simulink model "robot_ctc"  (R2019b)
settings: Solver=FixedStepAuto  StartTime=0.0  StopTime=20  FixedStep=0.001  RelTol=1e-3
InitFcn:
  | l1 = 0.26;
  | l2 = 0.26;
  | lc1 = 0.0983;
  | lc2 = 0.0229;
  | m1 = 6.5225;
  | m2 = 2.0458;
  | I1 = 0.1213;
  | I2 = 0.0116;
  | g = 9.81;
  | 
  | q0 = [pi/2, pi/6];
  | dq0 = [0, 0];
  | 
  | Kv = [10, 0; 0, 10];
  | Kp = [10, 0; 0, 10];
settings Model: Creator=jgakl

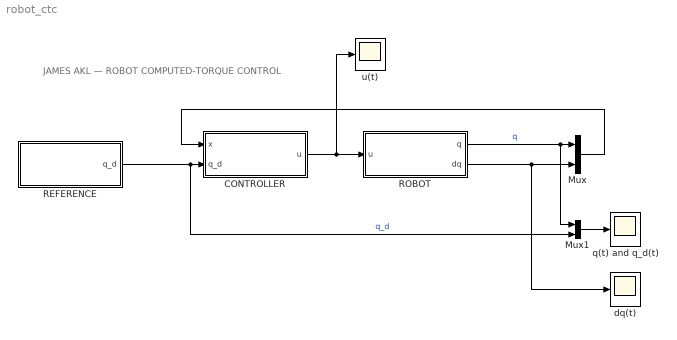
== system robot_ctc ==
  note: JAMES AKL — ROBOT COMPUTED-TORQUE CONTROL
  CONTROLLER : Subsystem
  Mux : Mux  Inputs=2
  Mux1 : Mux  Inputs=2
  REFERENCE : Subsystem
  ROBOT : Subsystem
  dq(t) : Scope
  q(t) and q_d(t) : Scope
  u(t) : Scope
  wires:
  CONTROLLER/1(u) -> u(t)/1, ROBOT/1(u)
  ROBOT/1(q) -> Mux1/1, Mux/1  "q"
  ROBOT/2(dq) -> dq(t)/1, Mux/2
  Mux/1 -> CONTROLLER/1(x)
  REFERENCE/1(q_d) -> CONTROLLER/2(q_d), Mux1/2  "q_d"
  Mux1/1 -> q(t) and q_d(t)/1

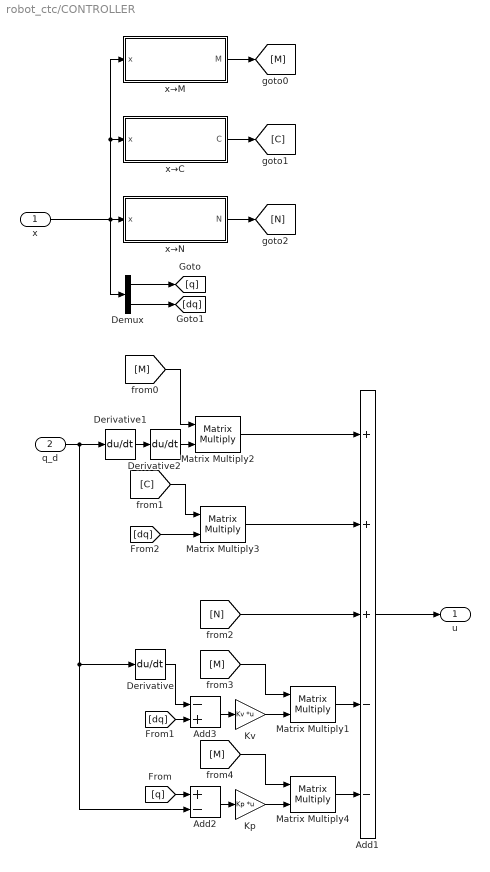
== system robot_ctc/CONTROLLER ==
  x : Inport
  q_d : Inport  Port=2
  Add1 : Sum  Inputs=+++--
  Add2 : Sum  Inputs=+-
  Add3 : Sum  Inputs=-+
  Demux : Demux  Outputs=2
  Derivative : Derivative
  Derivative1 : Derivative
  Derivative2 : Derivative
  Kp : Gain  Gain=Kp  Multiplication=Matrix(K*u) (u vector)
  Kv : Gain  Gain=Kv  Multiplication=Matrix(K*u) (u vector)
  Matrix Multiply{1..4} (4 alike) : Product  Multiplication=Matrix(*)
  x→C : Subsystem
  x→M : Subsystem
  x→N : Subsystem
  u : Outport
  wires:
  x→N/1(N) -> [N]
  x→C/1(C) -> [C]
  x/1 -> x→M/1(x), x→C/1(x), x→N/1(x), Demux/1
  x→M/1(M) -> [M]
  q_d/1 -> Derivative1/1, Derivative/1, Add2/2
  [M] -> Matrix Multiply2/1
  Matrix Multiply2/1 -> Add1/1
  Derivative/1 -> Add3/1
  [C] -> Matrix Multiply3/1
  Matrix Multiply3/1 -> Add1/2
  [N] -> Add1/3
  Derivative1/1 -> Derivative2/1
  Derivative2/1 -> Matrix Multiply2/2
  Demux/1 -> [q]
  Demux/2 -> [dq]
  [q] -> Add2/1
  [dq] -> Add3/2
  Add3/1 -> Kv/1
  Add2/1 -> Kp/1
  Kp/1 -> Matrix Multiply4/2
  Add1/1 -> u/1
  Kv/1 -> Matrix Multiply1/2
  Matrix Multiply1/1 -> Add1/4
  [M] -> Matrix Multiply1/1
  [M] -> Matrix Multiply4/1
  Matrix Multiply4/1 -> Add1/5
  [dq] -> Matrix Multiply3/2

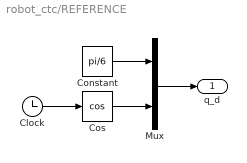
== system robot_ctc/REFERENCE ==
  Clock : Clock
  Constant : Constant  Value=pi/6
  Cos : Trigonometry  Operator=cos
  Mux : Mux  Inputs=2
  q_d : Outport
  wires:
  Clock/1 -> Cos/1
  Constant/1 -> Mux/1
  Mux/1 -> q_d/1
  Cos/1 -> Mux/2

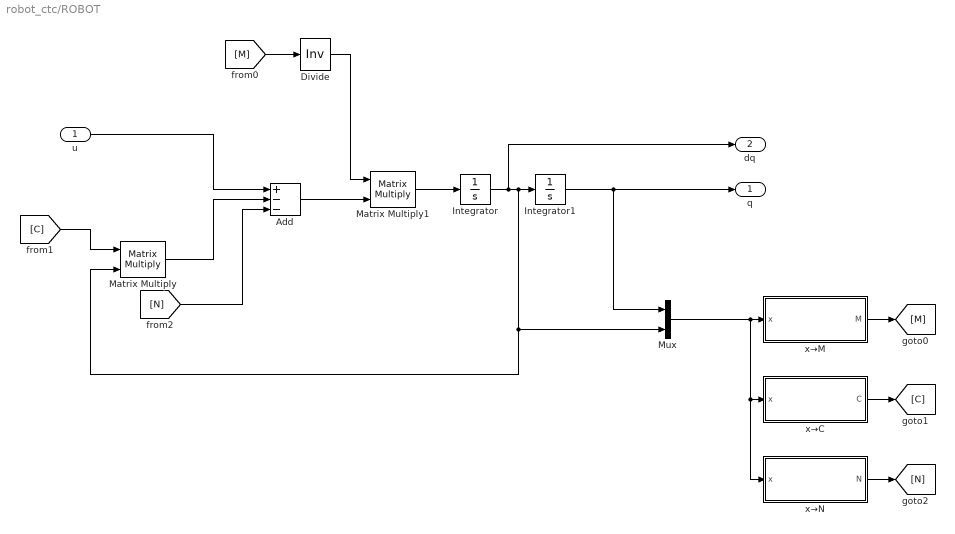
== system robot_ctc/ROBOT ==
  u : Inport
  Add : Sum  Inputs=+--
  Divide : Product  Inputs=/  Multiplication=Matrix(*)
  Integrator : Integrator  InitialCondition=dq0
  Integrator1 : Integrator  InitialCondition=q0
  Matrix Multiply : Product  Multiplication=Matrix(*)
  Matrix Multiply1 : Product  Multiplication=Matrix(*)
  Mux : Mux  Inputs=2
  x→C : Subsystem
  x→M : Subsystem
  x→N : Subsystem
  q : Outport
  dq : Outport  Port=2
  wires:
  [C] -> Matrix Multiply/1
  u/1 -> Add/1
  Matrix Multiply/1 -> Add/2
  [N] -> Add/3
  Add/1 -> Matrix Multiply1/2
  [M] -> Divide/1
  Divide/1 -> Matrix Multiply1/1
  Matrix Multiply1/1 -> Integrator/1
  Integrator/1 -> dq/1, Matrix Multiply/2, Mux/2, Integrator1/1
  Integrator1/1 -> Mux/1, q/1
  x→M/1(M) -> [M]
  x→C/1(C) -> [C]
  x→N/1(N) -> [N]
  Mux/1 -> x→N/1(x), x→C/1(x), x→M/1(x)

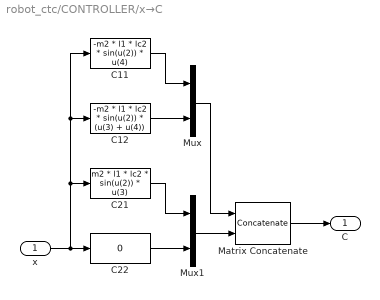
== system robot_ctc/CONTROLLER/x→C ==
  x : Inport
  C11 : Fcn  Expr=-m2 * l1 * lc2 * sin(u(2)) * u(4)
  C12 : Fcn  Expr=-m2 * l1 * lc2 * sin(u(2)) * (u(3) + u(4))
  C21 : Fcn  Expr=m2 * l1 * lc2 * sin(u(2)) * u(3)
  C22 : Fcn  Expr=0
  Matrix Concatenate : Concatenate  Mode=Multidimensional array  ConcatenateDimension=2
  Mux : Mux  Inputs=2
  Mux1 : Mux  Inputs=2
  C : Outport
  wires:
  Matrix Concatenate/1 -> C/1
  Mux1/1 -> Matrix Concatenate/2
  Mux/1 -> Matrix Concatenate/1
  C21/1 -> Mux1/1
  C22/1 -> Mux1/2
  C11/1 -> Mux/1
  C12/1 -> Mux/2
  x/1 -> C12/1, C11/1, C21/1, C22/1

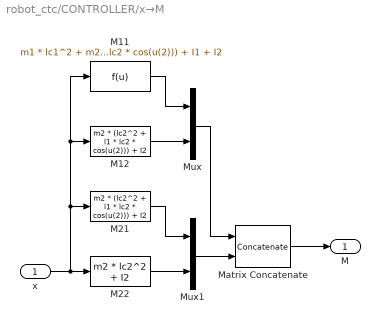
== system robot_ctc/CONTROLLER/x→M ==
  x : Inport
  M11 : Fcn  Expr=m1 * lc1^2 + m2 * (l1^2 + lc2^2 + 2 * l1 * lc2 * cos(u(2))) + I1 + I2
  M12 : Fcn  Expr=m2 * (lc2^2 + l1 * lc2 * cos(u(2))) + I2
  M21 : Fcn  Expr=m2 * (lc2^2 + l1 * lc2 * cos(u(2))) + I2
  M22 : Fcn  Expr=m2 * lc2^2 + I2
  Matrix Concatenate : Concatenate  Mode=Multidimensional array  ConcatenateDimension=2
  Mux : Mux  Inputs=2
  Mux1 : Mux  Inputs=2
  M : Outport
  wires:
  Matrix Concatenate/1 -> M/1
  Mux1/1 -> Matrix Concatenate/2
  Mux/1 -> Matrix Concatenate/1
  M21/1 -> Mux1/1
  M22/1 -> Mux1/2
  M11/1 -> Mux/1
  M12/1 -> Mux/2
  x/1 -> M12/1, M11/1, M21/1, M22/1

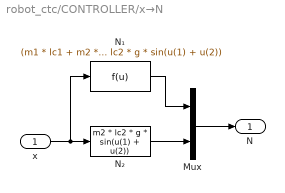
== system robot_ctc/CONTROLLER/x→N ==
  x : Inport
  Mux : Mux  Inputs=2
  N₂ : Fcn  Expr=m2 * lc2 * g * sin(u(1) + u(2))
  N︎₁ : Fcn  Expr=(m1 * lc1 + m2 * l1) * g * sin(u(1)) + m2 * lc2 * g * sin(u(1) + u(2))
  N : Outport
  wires:
  x/1 -> N₂/1, N︎₁/1
  N︎₁/1 -> Mux/1
  N₂/1 -> Mux/2
  Mux/1 -> N/1

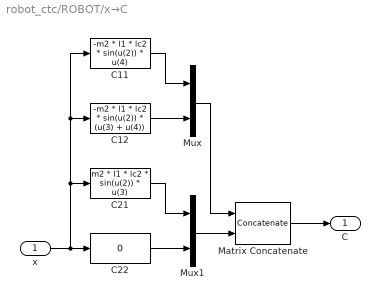
== system robot_ctc/ROBOT/x→C ==
  x : Inport
  C11 : Fcn  Expr=-m2 * l1 * lc2 * sin(u(2)) * u(4)
  C12 : Fcn  Expr=-m2 * l1 * lc2 * sin(u(2)) * (u(3) + u(4))
  C21 : Fcn  Expr=m2 * l1 * lc2 * sin(u(2)) * u(3)
  C22 : Fcn  Expr=0
  Matrix Concatenate : Concatenate  Mode=Multidimensional array  ConcatenateDimension=2
  Mux : Mux  Inputs=2
  Mux1 : Mux  Inputs=2
  C : Outport
  wires:
  Matrix Concatenate/1 -> C/1
  Mux1/1 -> Matrix Concatenate/2
  Mux/1 -> Matrix Concatenate/1
  C21/1 -> Mux1/1
  C22/1 -> Mux1/2
  C11/1 -> Mux/1
  C12/1 -> Mux/2
  x/1 -> C12/1, C11/1, C21/1, C22/1

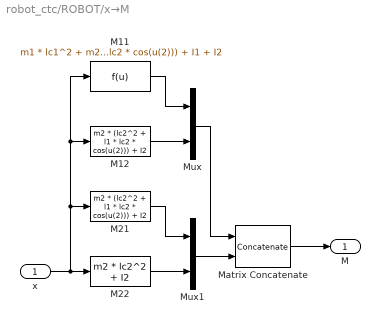
== system robot_ctc/ROBOT/x→M ==
  x : Inport
  M11 : Fcn  Expr=m1 * lc1^2 + m2 * (l1^2 + lc2^2 + 2 * l1 * lc2 * cos(u(2))) + I1 + I2
  M12 : Fcn  Expr=m2 * (lc2^2 + l1 * lc2 * cos(u(2))) + I2
  M21 : Fcn  Expr=m2 * (lc2^2 + l1 * lc2 * cos(u(2))) + I2
  M22 : Fcn  Expr=m2 * lc2^2 + I2
  Matrix Concatenate : Concatenate  Mode=Multidimensional array  ConcatenateDimension=2
  Mux : Mux  Inputs=2
  Mux1 : Mux  Inputs=2
  M : Outport
  wires:
  Matrix Concatenate/1 -> M/1
  Mux1/1 -> Matrix Concatenate/2
  Mux/1 -> Matrix Concatenate/1
  M21/1 -> Mux1/1
  M22/1 -> Mux1/2
  M11/1 -> Mux/1
  M12/1 -> Mux/2
  x/1 -> M12/1, M11/1, M21/1, M22/1

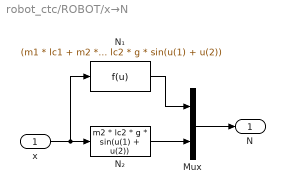
== system robot_ctc/ROBOT/x→N ==
  x : Inport
  Mux : Mux  Inputs=2
  N₂ : Fcn  Expr=m2 * lc2 * g * sin(u(1) + u(2))
  N︎₁ : Fcn  Expr=(m1 * lc1 + m2 * l1) * g * sin(u(1)) + m2 * lc2 * g * sin(u(1) + u(2))
  N : Outport
  wires:
  x/1 -> N₂/1, N︎₁/1
  N︎₁/1 -> Mux/1
  N₂/1 -> Mux/2
  Mux/1 -> N/1
